simulink model "Passive_System_Model"  (R2024a)
settings: Solver=VariableStepAuto  StartTime=0.0  StopTime=15  RelTol=1e-3
settings Model: Creator=LENOVO  LastModifiedBy=Jashwanth
settings SolverCC: AlgebraicLoopSolver=TrustRegion
settings DataIOCC: ReturnWorkspaceOutputs=off
settings DebuggingCC: UnconnectedInputMsg=warning  UnconnectedOutputMsg=warning  UnconnectedLineMsg=warning  ArithmeticOperatorsInVariantConditions=warning
settings ModelReferenceCC: EnableRefExpFcnMdlSchedulingChecks=on
settings SFSimCC: SimUseLocalCustomCode=off  CustomCodeUndefinedFunction=UseInterfaceOnly
settings RTWCC: RTWUseLocalCustomCode=off  GPUComputeCapability=3.5

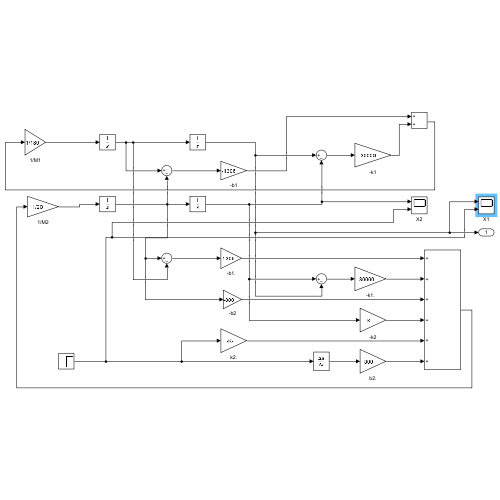
[thumbnail: Simulink's stored preview of the top-level diagram]
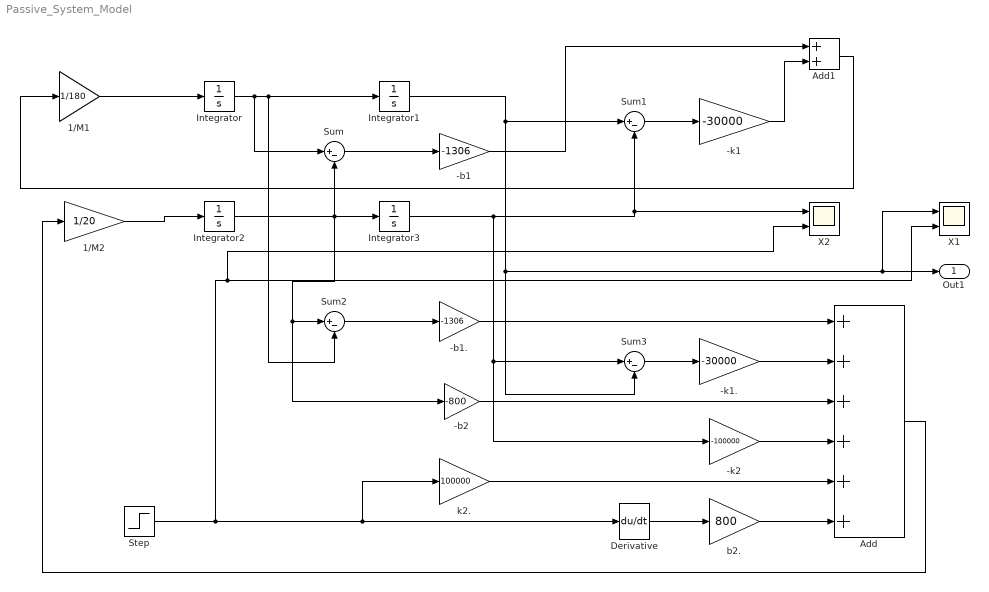
== system Passive_System_Model ==
  -b1 : Gain  Gain=-1306
  -b1. : Gain  Gain=-1306
  -b2 : Gain  Gain=-800
  -k1 : Gain  Gain=-30000
  -k1. : Gain  Gain=-30000
  -k2 : Gain  Gain=-100000
  1/M1 : Gain  Gain=1/180
  1/M2 : Gain  Gain=1/20
  Add : Sum  Inputs=++++++
  Add1 : Sum
  Derivative : Derivative
  Integrator{,1..3} (4 alike) : Integrator
  Step : Step  Time=5  SampleTime=0
  Sum{,1..3} (4 alike) : Sum  Inputs=|+-
  X1 : Scope  NumInputPorts=2
  X2 : Scope  NumInputPorts=2
  b2. : Gain  Gain=800
  k2. : Gain  Gain=100000
  Out1 : Outport  VectorParamsAs1DForOutWhenUnconnected=off
  wires:
  1/M2/1 -> Integrator2/1
  Integrator3/1 -> Sum3/1, -k2/1, Sum1/2, X2/1
  Integrator2/1 -> Sum2/1, -b2/1, Sum/2, Integrator3/1
  Sum2/1 -> -b1./1
  Sum/1 -> -b1/1
  Integrator/1 -> Sum/1, Sum2/2, Integrator1/1
  -b1/1 -> Add1/1
  Sum3/1 -> -k1./1
  k2./1 -> Add/5
  Add/1 -> 1/M2/1
  -k1/1 -> Add1/2
  -k1./1 -> Add/2
  -k2/1 -> Add/4
  Derivative/1 -> b2./1
  -b2/1 -> Add/3
  -b1./1 -> Add/1
  Integrator1/1 -> Sum1/1, X1/1, Out1/1, Sum3/2
  Sum1/1 -> -k1/1
  Step/1 -> X2/2, X1/2, Derivative/1, k2./1
  b2./1 -> Add/6
  1/M1/1 -> Integrator/1
  Add1/1 -> 1/M1/1
